simulink model "two_water_tanks"  (R2022b)
settings: Solver=ode45  StartTime=0.0  StopTime=250  RelTol=1e-3  EnableMultiTasking=on
PreLoadFcn:
  | % Parameters
  | A = 4;      % Area of bottom of tank [m^2]
  | hmax = 2;   % Height of tank [m]
  | R = 5;      % Resistance of exit [(kg*m)^-1/2]
  | W_in = 100; % Water inflow rate [kg/s]
  | rho = 1000; % Density of water [kg/m^3]
  | g = 9.81;   % Gravitational acceleration [m/s^2]
  | h0 = 0;     % Initial water height [m]
libraries: simulink x2
settings Model: Creator=nicholas  LastModifiedBy=bensweet
settings SolverCC: AlgebraicLoopSolver=TrustRegion
settings DataIOCC: LimitDataPoints=on  SaveFormat=Array  ReturnWorkspaceOutputs=off  SignalLoggingName=sigsOut
settings OptimizationCC: BooleanDataType=off  OptimizeBlockIOStorage=off  BufferReuse=off  GlobalBufferReuse=off  ExpressionFolding=off  ExpressionDepthLimit=2147483647  LocalBlockOutputs=off  InitFltsAndDblsToZero=on  LifeSpan=inf  OptimizeDataStoreBuffers=off  BusAssignmentInplaceUpdate=off
settings DebuggingCC: CheckExecutionContextPreStartOutputMsg=on  UnconnectedInputMsg=warning  UnconnectedOutputMsg=warning  UnconnectedLineMsg=warning  PregeneratedLibrarySubsystemCodeDiagnostic=none  SFMachineParentedDataDiag=warning
settings HardwareCC: ProdBitPerPointer=32  ProdBitPerSizeT=32  ProdBitPerPtrDiffT=32  ProdLargestAtomicFloat=None  ProdIntDivRoundTo=Undefined  ProdEndianess=Unspecified  ProdWordSize=32  ProdHWDeviceType=32-bit Generic  TargetUnknown=on
settings ModelReferenceCC: EnableRefExpFcnMdlSchedulingChecks=on  PropagateSignalLabelsOutOfModel=off
settings SFSimCC: SimUseLocalCustomCode=off
settings RTWCC: RTWUseLocalCustomCode=off  DLArmComputeVersion=19.05
settings CodeAppCC: StateflowObjectComments=on
settings GRTTargetCC: TargetFcnLib=ansi_tfl_tmw.mat  TargetLangStandard=C89/C90 (ANSI)  CombineOutputUpdateFcns=off  GRTInterface=on
settings ConfigComp: CovMetricSettings=dw  CovSaveCumulativeToWorkspaceVar=on  CovSaveSingleToWorkspaceVar=on  CovExternalEMLEnable=off  CovSFcnEnable=off

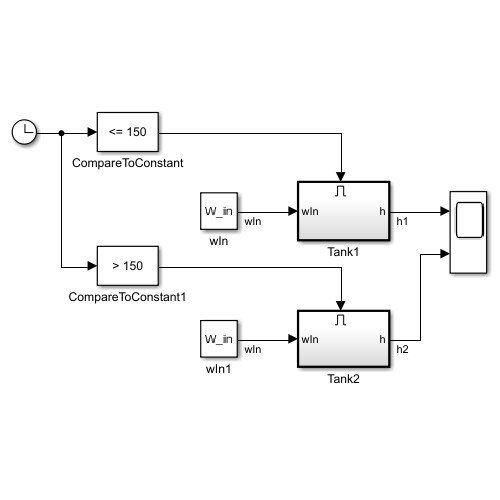
[thumbnail: Simulink's stored preview of the top-level diagram]
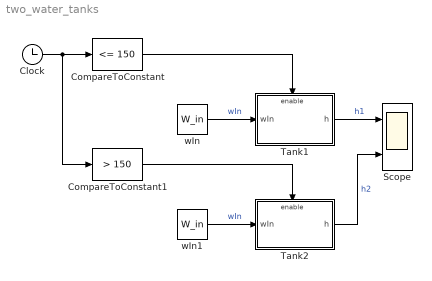
== system two_water_tanks ==
  Clock : Clock
  CompareToConstant : simulink/Logic and Bit Operations/Compare To Constant  relop=<=  const=150  OutDataTypeStr=uint8
  CompareToConstant1 : simulink/Logic and Bit Operations/Compare To Constant  relop=>  const=150  OutDataTypeStr=uint8
  Scope : Scope  NumInputPorts=2
  Tank1 : Subsystem
  Tank2 : Subsystem
  wIn : Constant  Value=W_in
  wIn1 : Constant  Value=W_in
  wires:
  Tank1/1(h) -> Scope/1  "h1"
  wIn/1 -> Tank1/1(wIn)  "wIn"
  wIn1/1 -> Tank2/1(wIn)  "wIn"
  Tank2/1(h) -> Scope/2  "h2"
  Clock/1 -> CompareToConstant/1, CompareToConstant1/1
  CompareToConstant/1 -> Tank1/Enable
  CompareToConstant1/1 -> Tank2/Enable

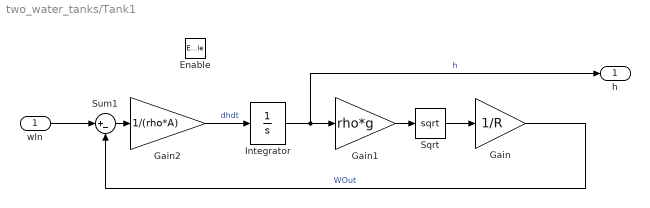
== system two_water_tanks/Tank1 ==
  wIn : Inport
  Enable : EnablePort
  Gain : Gain  Gain=1/R  SaturateOnIntegerOverflow=on  OutDataTypeStr=Inherit: Same as input  ParamDataTypeStr=Inherit: Same as input
  Gain1 : Gain  Gain=rho*g  SaturateOnIntegerOverflow=on  OutDataTypeStr=Inherit: Same as input  ParamDataTypeStr=Inherit: Same as input
  Gain2 : Gain  Gain=1/(rho*A)  SaturateOnIntegerOverflow=on  OutDataTypeStr=Inherit: Same as input  ParamDataTypeStr=Inherit: Same as input
  Integrator : Integrator  InitialCondition=h0  UpperSaturationLimit=hmax  LowerSaturationLimit=0
      settings: AttributesFormatString=IC: %<InitialCondition>
  Sqrt : Sqrt
  Sum1 : Sum  Inputs=|+-  InputSameDT=on  SaturateOnIntegerOverflow=on  OutDataTypeStr=Inherit: Same as first input
  h : Outport  InitialOutput=h0  VectorParamsAs1DForOutWhenUnconnected=off
  wires:
  Integrator/1 -> Gain1/1, h/1  "h"
  Gain1/1 -> Sqrt/1
  Sqrt/1 -> Gain/1
  Gain2/1 -> Integrator/1  "dhdt"
  Sum1/1 -> Gain2/1
  Gain/1 -> Sum1/2  "WOut"
  wIn/1 -> Sum1/1

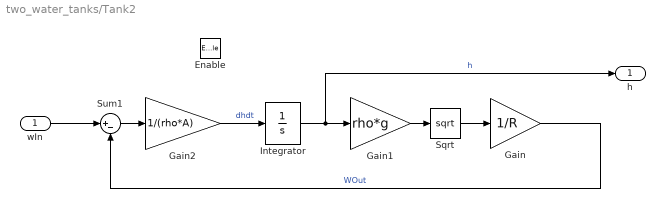
== system two_water_tanks/Tank2 ==
  wIn : Inport
  Enable : EnablePort
  Gain : Gain  Gain=1/R  SaturateOnIntegerOverflow=on  OutDataTypeStr=Inherit: Same as input  ParamDataTypeStr=Inherit: Same as input
  Gain1 : Gain  Gain=rho*g  SaturateOnIntegerOverflow=on  OutDataTypeStr=Inherit: Same as input  ParamDataTypeStr=Inherit: Same as input
  Gain2 : Gain  Gain=1/(rho*A)  SaturateOnIntegerOverflow=on  OutDataTypeStr=Inherit: Same as input  ParamDataTypeStr=Inherit: Same as input
  Integrator : Integrator  InitialCondition=h0  UpperSaturationLimit=hmax  LowerSaturationLimit=0
      settings: AttributesFormatString=IC: %<InitialCondition>
  Sqrt : Sqrt
  Sum1 : Sum  Inputs=|+-  InputSameDT=on  SaturateOnIntegerOverflow=on  OutDataTypeStr=Inherit: Same as first input
  h : Outport  InitialOutput=h0  VectorParamsAs1DForOutWhenUnconnected=off
  wires:
  wIn/1 -> Sum1/1
  Gain/1 -> Sum1/2  "WOut"
  Sum1/1 -> Gain2/1
  Gain2/1 -> Integrator/1  "dhdt"
  Sqrt/1 -> Gain/1
  Gain1/1 -> Sqrt/1
  Integrator/1 -> h/1, Gain1/1  "h"
